simulink model "VB_RIFKF_UWB_INS25"  (R2023a)
settings: Solver=FixedStepAuto  StartTime=0.0  StopTime=500  FixedStep=0.01  RelTol=1e-3
InitFcn:
  | resilient_initNavigation1216;
  | init_param;
  | param_bias;
undefined symbols (not defined in the file or in its folder): dt, g0, gam0_rad, ISUS_flag, lp_GPS_sample_time, lp_Lidar_knoise, lp_Lidar_max, lp_Lidar_min, lp_Lidar_sample_time, lp_Lidar_seed, lp_UWB_knoise, lp_UWB_sample_time, lp_UWB_seed, lp_UWB_XY_max, lp_UWB_XY_min, magnitude, p, P0, P0_RIEKF, param, pd0, pe0, phi0_rad, pn0, psi, psi0_rad, state_dim, vd0, ve0, vn0
libraries: simulink_extras x108, simulink x89, dspstat3 x74, sharedtransform x61, matrix_library x11, sharedTrackingLibrary x8, aerolibconvert2 x5, aerolibtransform2 x5, dspfactors x3
(part 20 of 29)

== system VB_RIFKF_UWB_INS25/ISUS_RIEKF3/Error State Kalman Filter M4/Extended Kalman Filter M1/Correct M1 ==
  yMeas : Inport  SampleTime=SampleTime
  R : Inport  Port=2  SampleTime=SampleTime
  uMeas : Inport  Port=3  SampleTime=SampleTime
  uBlockOrdering : Inport  Port=4  SampleTime=SampleTime
  H : Inport  Port=5  SampleTime=SampleTime
  pk_1 : Inport  Port=6
  Enable : EnablePort
  Cholesky Factorization : dspfactors/Cholesky Factorization  errmode=Warning
  Correct : MATLAB Function  TreatAsAtomicUnit=on
  Data Store Read : DataStoreRead  DataStoreName=x  IndexOptions=Index vector (dialog)  Indices=1  OutputSizes=1
  Data Store Read1 : DataStoreRead  DataStoreName=P  IndexOptions=Index vector (dialog)  Indices=1  OutputSizes=1
  Data Store Write2 : DataStoreWrite  Commented=on  DataStoreName=x  IndexOptions=Index vector (dialog)  Indices=1  OutputSizes=1
  Data Store Write3 : DataStoreWrite  Commented=on  DataStoreName=P  IndexOptions=Index vector (dialog)  Indices=1  OutputSizes=1
  Data Store WriteP : DataStoreWrite  DataStoreName=P  IndexOptions=Index vector (dialog)  Indices=1  OutputSizes=1
  Data Store WriteX : DataStoreWrite  DataStoreName=x  IndexOptions=Index vector (dialog)  Indices=1  OutputSizes=1
  MATLAB Function : MATLAB Function  TreatAsAtomicUnit=on
  R1 : InportShadow  Port=2  SampleTime=SampleTime
  RegisterSimulinkFcn : S-Function  FunctionName=ekfukfRegisterSimulinkFcn  Parameters=int32(3), 1, pM.HasAdditiveNoise, SampleTime, DataType, SLFcnsToRegister  SFunctionDeploymentMode=off  EnableBusSupport=off
  Scope : Scope
  Subsystem2 : Subsystem
  innovation calculation : Subsystem
  yMeas1 : InportShadow  SampleTime=SampleTime
  yBlockOrdering : Outport  VectorParamsAs1DForOutWhenUnconnected=off
  Sk : Outport  Port=2  VectorParamsAs1DForOutWhenUnconnected=off
  m_innov : Outport  Port=3  VectorParamsAs1DForOutWhenUnconnected=off
  wires:
  MATLAB Function/1(y) -> Subsystem2/1(Pk_1_ISIU)
  Cholesky Factorization/1 -> MATLAB Function/1(u)
  pk_1/1 -> Cholesky Factorization/1
  Correct/2(P) -> Data Store WriteP/1
  Data Store Read1/1 -> Subsystem2/2(Pk_2)
  Subsystem2/1(y1) -> Correct/2("P "), innovation calculation/1(Pk/k_1)
  Data Store Read/1 -> RegisterSimulinkFcn/1, Correct/1(x)
  H/1 -> innovation calculation/5(H)
  innovation calculation/1(Sk) -> Sk/1
  innovation calculation/2(m_innov) -> m_innov/1
  R1/1 -> innovation calculation/4(R)
  yMeas1/1 -> innovation calculation/2(yMeas)
  yMeas/1 -> Correct/3(yMeas), RegisterSimulinkFcn/2, Scope/1
  R/1 -> Correct/4(R), RegisterSimulinkFcn/3
  Correct/1(xNew) -> Data Store WriteX/1, innovation calculation/3(X)
  Correct/3(blockOrdering) -> yBlockOrdering/1
  uBlockOrdering/1 -> Correct/6("blockOrdering ")
  uMeas/1 -> Correct/5(uMeas)

== system VB_RIFKF_UWB_INS25/ISUS_RIEKF3/Error State Kalman Filter M4/Extended Kalman Filter M1/Output ==
  uBlockOrdering : Inport
  Data Store Read : DataStoreRead  DataStoreName=x  IndexOptions=Index vector (dialog)  Indices=1  OutputSizes=1
  Data Store Read1 : DataStoreRead  DataStoreName=P  IndexOptions=Index vector (dialog)  Indices=1  OutputSizes=1
  MATLAB Function : MATLAB Function  TreatAsAtomicUnit=on
  x : Outport  VectorParamsAs1DForOutWhenUnconnected=off
  P : Outport  Port=2  VectorParamsAs1DForOutWhenUnconnected=off
  yBlockOrdering : Outport  Port=3  VectorParamsAs1DForOutWhenUnconnected=off
  wires:
  MATLAB Function/1(P) -> P/1
  Data Store Read1/1 -> MATLAB Function/1(S)
  Data Store Read/1 -> x/1
  uBlockOrdering/1 -> yBlockOrdering/1

== system VB_RIFKF_UWB_INS25/ISUS_RIEKF3/Error State Kalman Filter M4/Extended Kalman Filter M1/Predict ==
  Q : Inport  SampleTime=SampleTime
  uState : Inport  Port=2  SampleTime=SampleTime
  uBlockOrdering : Inport  Port=3  SampleTime=SampleTime
  Data Store Read1 : DataStoreRead  Commented=on  DataStoreName=feedback_flag_18dim  IndexOptions=Index vector (dialog)  Indices=1  OutputSizes=1
  Data Store Write : DataStoreWrite  DataStoreName=P  IndexOptions=Index vector (dialog)  Indices=1  OutputSizes=1
  Data Store Write1 : DataStoreWrite  DataStoreName=x  IndexOptions=Index vector (dialog)  Indices=1  OutputSizes=1
  Data Store WriteX : DataStoreWrite  DataStoreName=x  IndexOptions=Index vector (dialog)  Indices=1  OutputSizes=1
  Data Store ReadP : DataStoreRead  DataStoreName=P  IndexOptions=Index vector (dialog)  Indices=1  OutputSizes=1
  Data Store ReadX : DataStoreRead  DataStoreName=x  IndexOptions=Index vector (dialog)  Indices=1  OutputSizes=1
  If : If  Commented=on  IfExpression=u1 == 1  ShowElse=off
  If Action Subsystem : Subsystem  Commented=on  TreatAsAtomicUnit=on
  Predict : MATLAB Function  TreatAsAtomicUnit=on
  RegisterSimulinkFcn : S-Function  FunctionName=ekfukfRegisterSimulinkFcn  Parameters=int32(2), 0, pS.HasAdditiveNoise, SampleTime, DataType, SLFcnsToRegister  SFunctionDeploymentMode=off  EnableBusSupport=off
  Zero : Constant  Value=zeros(state_dim,1)  OutDataTypeStr=Inherit: Inherit via back propagation
  wires:
  Data Store ReadP/1 -> Predict/2("P ")
  Predict/2(P) -> Data Store Write/1
  Q/1 -> Predict/3(Q), RegisterSimulinkFcn/2
  Predict/1(xNew) -> Data Store WriteX/1
  Data Store ReadX/1 -> Predict/1(x), RegisterSimulinkFcn/1
  uBlockOrdering/1 -> Predict/5(unused)
  uState/1 -> Predict/4(uState)
  Data Store Read1/1 -> If/1
  If/1 -> If Action Subsystem/Action
  Zero/1 -> Data Store Write1/1

== system VB_RIFKF_UWB_INS25/ISUS_RIEKF3/Error State Kalman Filter M4/Extended Kalman Filter M1/innovation calculation ==
  Pk/k_1 : Inport
  yMeas : Inport  Port=2
  X : Inport  Port=3
  R : Inport  Port=4
  H : Inport  Port=5
  Add : Sum
  Add1 : Sum  Inputs=+-
  MATLAB Function : MATLAB Function  TreatAsAtomicUnit=on
  Product : Product  Inputs=3  Multiplication=Matrix(*)
  Product1 : Product  Multiplication=Matrix(*)
  Scope1 : Scope
  Scope2 : Scope
  Transpose : Math  Operator=transpose
  Sk : Outport
  m_innov : Outport  Port=2
  wires:
  MATLAB Function/1(y) -> Product/2
  Product/1 -> Add/1
  Transpose/1 -> Product/3
  R/1 -> Add/2
  Pk/k_1/1 -> MATLAB Function/1(u)
  yMeas/1 -> Add1/1
  H/1 -> Product1/1, Product/1, Transpose/1
  X/1 -> Product1/2, Scope2/1
  Product1/1 -> Add1/2
  Add/1 -> Sk/1  "S"
  Add1/1 -> m_innov/1, Scope1/1

== system VB_RIFKF_UWB_INS25/ISUS_RIEKF3/Error State Kalman Filter M4/Simulink Function - State Transition/Cal Phi ==
  Rbn : Inport
  vn : Inport  Port=2
  pn : Inport  Port=3
  Constant : Constant  Value=dt
  MATLAB Function1 : MATLAB Function  TreatAsAtomicUnit=on
  Reshape : Reshape  OutputDimensionality=Column vector (2-D)
  Reshape1 : Reshape  OutputDimensionality=Column vector (2-D)
  Phi : Outport
  wires:
  Reshape1/1 -> MATLAB Function1/2(pn)
  Reshape/1 -> MATLAB Function1/1(vn)
  pn/1 -> Reshape1/1
  vn/1 -> Reshape/1
  Rbn/1 -> MATLAB Function1/3(Rbn)
  MATLAB Function1/1(Phi) -> Phi/1
  Constant/1 -> MATLAB Function1/4(dt)

== system VB_RIFKF_UWB_INS25/ISUS_RIEKF3/Error State Kalman Filter M4/Simulink Function - State Transition1/Cal Phi ==
  Rbn : Inport
  vn : Inport  Port=2
  pn : Inport  Port=3
  Constant : Constant  Value=dt  OutDataTypeStr=single
  MATLAB Function1 : MATLAB Function  TreatAsAtomicUnit=on
  Reshape : Reshape  OutputDimensionality=Column vector (2-D)
  Reshape1 : Reshape  OutputDimensionality=Column vector (2-D)
  Phi : Outport
  wires:
  Constant/1 -> MATLAB Function1/4(dt)
  MATLAB Function1/1(Phi) -> Phi/1
  Rbn/1 -> MATLAB Function1/3(Rbn)
  vn/1 -> Reshape/1
  pn/1 -> Reshape1/1
  Reshape/1 -> MATLAB Function1/1(vn)
  Reshape1/1 -> MATLAB Function1/2(pn)

== system VB_RIFKF_UWB_INS25/ISUS_RIEKF3/Error State Kalman Filter M4/bak/Simulink Function - GPS Measurements1 ==
  DCM_b_n : Inport
  DynamicMeasurementFcn_Dyn : TriggerPort  TriggerType=function-call  IsSimulinkFunction=on  FunctionName=DynamicMeasurementFcn_Dyn  VariantControl=Variant
  Add : Sum  Commented=on
  Add1 : Sum
  Constant : Constant  Commented=on  Value=dt  OutDataTypeStr=single
  Constant6 : Constant  Value=[zeros(3,3),eye(3),zeros(3,12);zeros(3,15),eye(3)]  OutDataTypeStr=single
  Data Type Conversion6 : DataTypeConversion  Commented=on  OutDataTypeStr=single  SaturateOnIntegerOverflow=off  RndMeth=Floor
  From7 : From  Commented=on  GotoTag=DCM_b_n
  Goto : Goto  Commented=on  GotoTag=DCM_b_n
  MATLAB Function1 : MATLAB Function  Commented=on  TreatAsAtomicUnit=on
  Product : Product  Commented=on  Multiplication=Matrix(*)
  Product1 : Product  Multiplication=Matrix(*)
  x : ArgIn  DisableCoverage=on  OutDataTypeStr=single  PortDimensions=18  ArgumentName=x
  v : ArgIn  DisableCoverage=on  Port=2  OutDataTypeStr=single  PortDimensions=6  ArgumentName=v
  y : ArgOut  DisableCoverage=on  OutDataTypeStr=single  PortDimensions=6  ArgumentName=y
  wires:
  x/1 -> Product1/2
  Constant6/1 -> Product1/1
  Product1/1 -> Add1/1
  v/1 -> Add1/2
  Add1/1 -> y/1
  Data Type Conversion6/1 -> Product/1
  DCM_b_n/1 -> Goto/1
  Constant/1 -> MATLAB Function1/2(dt)
  From7/1 -> MATLAB Function1/1(Cbn)
  MATLAB Function1/1(H) -> Data Type Conversion6/1
  Product/1 -> Add/1

== system VB_RIFKF_UWB_INS25/ISUS_RIEKF3/Error State Kalman Filter M4/bak/Simulink Function - GPS Measurements2 ==
  ZUPTMeasurementFcn2 : TriggerPort  TriggerType=function-call  IsSimulinkFunction=on  FunctionName=ZUPTMeasurementFcn2  VariantControl=Variant
  Add : Sum
  Constant6 : Constant  Value=[zeros(3,3),eye(3),zeros(3,12)]  OutDataTypeStr=single
  Product : Product  Multiplication=Matrix(*)
  x : ArgIn  DisableCoverage=on  OutDataTypeStr=single  PortDimensions=18  ArgumentName=x
  v : ArgIn  DisableCoverage=on  Port=2  OutDataTypeStr=single  PortDimensions=3  ArgumentName=v
  y : ArgOut  DisableCoverage=on  OutDataTypeStr=single  PortDimensions=3  ArgumentName=y
  wires:
  v/1 -> Add/2
  Constant6/1 -> Product/1
  x/1 -> Product/2
  Product/1 -> Add/1
  Add/1 -> y/1

== system VB_RIFKF_UWB_INS25/ISUS_RIEKF3/Error State Kalman Filter M4/bak/Simulink Function - State Transition Jacobian ==
  DCM_b_n : Inport
  vn : Inport  Port=2
  pn : Inport  Port=3
  stateTransitionJacobianFcn_Dyn : TriggerPort  TriggerType=function-call  IsSimulinkFunction=on  FunctionName=stateTransitionJacobianFcn_Dyn  VariantControl=Variant
  Cal Phi1 : Subsystem
  Constant : Constant  Value=0.01  OutDataTypeStr=single
  Data Type Conversion1 : DataTypeConversion  OutDataTypeStr=single  SaturateOnIntegerOverflow=off  RndMeth=Floor
  Data Type Conversion6 : DataTypeConversion  OutDataTypeStr=single  SaturateOnIntegerOverflow=off  RndMeth=Floor
  MATLAB Function1 : MATLAB Function  TreatAsAtomicUnit=on
  Product : Product  Multiplication=Matrix(*)
  Terminator : Terminator
  Terminator1 : Terminator
  Transpose : Math  Operator=transpose
  x : ArgIn  DisableCoverage=on  OutDataTypeStr=single  PortDimensions=15  ArgumentName=x
  w : ArgIn  Port=2  OutDataTypeStr=single  PortDimensions=12  ArgumentName=w
  A : ArgOut  DisableCoverage=on  OutDataTypeStr=single  PortDimensions=[15 15]  ArgumentName=A
  G : ArgOut  Port=2  OutDataTypeStr=single  PortDimensions=[15 12]  ArgumentName=G
  wires:
  Data Type Conversion1/1 -> Product/2
  Product/1 -> G/1
  [pn] -> MATLAB Function1/3(pn)
  [vn] -> MATLAB Function1/2(vn)
  Data Type Conversion6/1 -> A/1, Product/1
  Constant/1 -> MATLAB Function1/4(dt)
  Transpose/1 -> MATLAB Function1/1(Rbn)
  [DCM_b_n] -> Transpose/1
  [DCM_b_n] -> Cal Phi1/1(Rbn)
  [pn] -> Cal Phi1/3(pn)
  [vn] -> Cal Phi1/2(vn)
  vn/1 -> [vn]
  pn/1 -> [pn]
  DCM_b_n/1 -> [DCM_b_n]
  Cal Phi1/1(Phi) -> Data Type Conversion6/1
  w/1 -> Terminator1/1
  x/1 -> Terminator/1
  MATLAB Function1/1(G) -> Data Type Conversion1/1

== system VB_RIFKF_UWB_INS25/ISUS_RIEKF3/INS propogation/Init_PVQ/Horizontal_attitude ==
  note: gamma
  note: fai
  accl_mean_B_m/s_LPF : Inport  PortDimensions=3
  Magn_mean_B_guess_LPF : Inport  Port=2
  Enable : EnablePort
  Add : Sum  Commented=on  Inputs=+-
  Add1 : Sum
  Add2 : Sum
  Asin : Trigonometry  Operator=asin
  Atan2 : Trigonometry  Commented=on  Operator=atan2
  Data Type Conversion : DataTypeConversion  SaturateOnIntegerOverflow=off  RndMeth=Floor
  Deal with zero : Subsystem
  Degrees to Radians : simulink_extras/Transformations/Degrees to Radians  Commented=on
  Degrees to Radians1 : simulink_extras/Transformations/Degrees to Radians
  Demux : Demux  Outputs=3
  Display : Display
  Divide : Product  Inputs=*/  OutDataTypeStr=single
  Gain1 : Gain  Gain=-1
  Gain2 : Gain  Gain=-1
  Magnetic declination : Constant  Commented=on  Value=param.fusion.magDeclDeg  OutDataTypeStr=single
  Magnetic declination1 : Constant  Value=param.control.MagnheadingCorrection  OutDataTypeStr=uint8
  Math Function : Math  Operator=magnitude^2  SignedPower=on
  Mux : Mux  Inputs=3
  Mux1 : Mux  Inputs=3
  Mux3 : Mux  Commented=on  Inputs=3
  Product : Product  Commented=on  Multiplication=Matrix(*)
  Quaternions to Direction Cosine Matrix : sharedtransform/Quaternions to  Direction Cosine Matrix  Commented=on  aMode=aMode
  Radians to Degrees : simulink_extras/Transformations/Radians to Degrees  Commented=on
  Rotation Angles to Quaternions : sharedtransform/Rotation Angles to Quaternions  rotationOrder=ZYX  aMode=aMode
  Rotation Angles to Quaternions1 : sharedtransform/Rotation Angles to Quaternions  Commented=on  rotationOrder=ZYX  aMode=aMode
  Scope : Scope
  Scope1 : Scope
  Selector : Selector  Commented=on  InputPortWidth=3  IndexOptions=Index vector (dialog)  Indices=[2]  OutputSizes=1
  Selector1 : Selector  Commented=on  InputPortWidth=3  IndexOptions=Index vector (dialog)  Indices=[1]  OutputSizes=1
  Sqrt : Sqrt
  Sum of Elements : Sum  Inputs=+
  Switch : Switch  Threshold=0.5  SaturateOnIntegerOverflow=off  InputSameDT=off
  Terminator : Terminator  Commented=on
  Transpose : Math  Commented=on  Operator=transpose  SignedPower=on
  Trigonometric Function1 : Trigonometry  Operator=atan2
  phi0_rad : Constant  Value=phi0_rad  OutDataTypeStr=single
  phi0_rad1 : Constant  Value=gam0_rad  OutDataTypeStr=single
  psi_zero : Constant  Value=psi  OutDataTypeStr=single
  psi_zero1 : Constant  Commented=on  Value=psi  OutDataTypeStr=single
  quat_0 : Outport  PortDimensions=4
  wires:
  Gain2/1 -> Add2/2
  phi0_rad1/1 -> Add2/1
  phi0_rad/1 -> Add1/1
  Asin/1 -> Add1/2
  Radians to Degrees/1 -> Display/1
  Data Type Conversion/1 -> Scope/1
  Switch/1 -> quat_0/1, Scope1/1
  Magnetic declination1/1 -> Switch/2, Data Type Conversion/1
  Degrees to Radians/1 -> Terminator/1
  Degrees to Radians1/1 -> Mux1/1
  Gain1/1 -> Mux/3, Trigonometric Function1/2
  Transpose/1 -> Product/1
  Mux3/1 -> Rotation Angles to Quaternions1/1
  Add/1 -> Mux3/1, Radians to Degrees/1  "psi_calbymag"
  Magnetic declination/1 -> Degrees to Radians/1
  Atan2/1 -> Add/2
  Selector/1 -> Atan2/1  "magE"
  Selector1/1 -> Atan2/2  "magN"
  Product/1 -> Selector1/1, Selector/1  "magNED"
  Magn_mean_B_guess_LPF/1 -> Product/2
  Quaternions to Direction Cosine Matrix/1 -> Transpose/1
  Add2/1 -> Mux1/3, Mux3/3
  Add1/1 -> Mux1/2, Mux3/2
  psi_zero/1 -> Degrees to Radians1/1
  Mux1/1 -> Rotation Angles to Quaternions/1
  Math Function/1 -> Sum of Elements/1
  Mux/1 -> Math Function/1
  Divide/1 -> Asin/1
  Sum of Elements/1 -> Sqrt/1
  Demux/3 -> Gain1/1
  Demux/2 -> Trigonometric Function1/1, Mux/1
  Demux/1 -> Mux/2, Divide/1
  Trigonometric Function1/1 -> Gain2/1
  Deal with zero/1(Out1) -> Divide/2
  Sqrt/1 -> Deal with zero/1(In1)
  accl_mean_B_m/s_LPF/1 -> Demux/1
  Rotation Angles to Quaternions/1 -> Switch/1, Switch/3

== system VB_RIFKF_UWB_INS25/ISUS_RIEKF3/INS propogation/Init_PVQ/Subsystem ==
  data : Inport
  Buffer : Buffer  N=50  V=49  OutputFrames=off
  Buffer1 : Buffer  N=50  V=49  OutputFrames=off
  Buffer2 : Buffer  N=50  V=49  ic=-g0  OutputFrames=off
  Demux : Demux  Outputs=3
  Mean4 : dspstat3/Mean  run=off  reset_popup=None  directionMode=Entire input  dimension=3  roiEnable=off  roiType=Rectangles  roiPortion=Entire ROI  roiOutput=Individual statistics for each ROI  roiFlag=off  roundingMode=Floor  overflowMode=off  outputDataTypeStr=Inherit: Same as accumulator  outputMin=[]  outputMax=[]  outputLastDataTypeStr=Inherit: Same as accumulator
  Mean5 : dspstat3/Mean  run=off  reset_popup=None  directionMode=Entire input  dimension=3  roiEnable=off  roiType=Rectangles  roiPortion=Entire ROI  roiOutput=Individual statistics for each ROI  roiFlag=off  roundingMode=Floor  overflowMode=off  outputDataTypeStr=Inherit: Same as accumulator  outputMin=[]  outputMax=[]  outputLastDataTypeStr=Inherit: Same as accumulator
  Mean6 : dspstat3/Mean  run=off  reset_popup=None  directionMode=Entire input  dimension=3  roiEnable=off  roiType=Rectangles  roiPortion=Entire ROI  roiOutput=Individual statistics for each ROI  roiFlag=off  roundingMode=Floor  overflowMode=off  outputDataTypeStr=Inherit: Same as accumulator  outputMin=[]  outputMax=[]  outputLastDataTypeStr=Inherit: Same as accumulator
  Scope : Scope  NumInputPorts=2
  Vector Concatenate : Concatenate  NumInputs=3
  mean_data : Outport
  wires:
  data/1 -> Demux/1, Scope/1
  Vector Concatenate/1 -> mean_data/1, Scope/2
  Mean4/1 -> Vector Concatenate/1
  Demux/3 -> Buffer2/1
  Buffer1/1 -> Mean5/1  "fby_buff"
  Demux/1 -> Buffer/1
  Buffer2/1 -> Mean6/1  "fbz_buff"
  Mean5/1 -> Vector Concatenate/2
  Buffer/1 -> Mean4/1  "fbx_buff"
  Demux/2 -> Buffer1/1
  Mean6/1 -> Vector Concatenate/3

== system VB_RIFKF_UWB_INS25/ISUS_RIEKF3/INS propogation/Init_PVQ/Subsystem1 ==
  data : Inport
  Buffer : Buffer  N=50  V=49  OutputFrames=off
  Buffer1 : Buffer  N=50  V=49  OutputFrames=off
  Buffer2 : Buffer  N=50  V=49  OutputFrames=off
  Demux : Demux  Outputs=3
  Mean4 : dspstat3/Mean  run=off  reset_popup=None  directionMode=Entire input  dimension=3  roiEnable=off  roiType=Rectangles  roiPortion=Entire ROI  roiOutput=Individual statistics for each ROI  roiFlag=off  roundingMode=Floor  overflowMode=off  outputDataTypeStr=Inherit: Same as accumulator  outputMin=[]  outputMax=[]  outputLastDataTypeStr=Inherit: Same as accumulator
  Mean5 : dspstat3/Mean  run=off  reset_popup=None  directionMode=Entire input  dimension=3  roiEnable=off  roiType=Rectangles  roiPortion=Entire ROI  roiOutput=Individual statistics for each ROI  roiFlag=off  roundingMode=Floor  overflowMode=off  outputDataTypeStr=Inherit: Same as accumulator  outputMin=[]  outputMax=[]  outputLastDataTypeStr=Inherit: Same as accumulator
  Mean6 : dspstat3/Mean  run=off  reset_popup=None  directionMode=Entire input  dimension=3  roiEnable=off  roiType=Rectangles  roiPortion=Entire ROI  roiOutput=Individual statistics for each ROI  roiFlag=off  roundingMode=Floor  overflowMode=off  outputDataTypeStr=Inherit: Same as accumulator  outputMin=[]  outputMax=[]  outputLastDataTypeStr=Inherit: Same as accumulator
  Vector Concatenate : Concatenate  NumInputs=3
  mean_data : Outport
  wires:
  Mean6/1 -> Vector Concatenate/3
  Demux/2 -> Buffer1/1
  Buffer/1 -> Mean4/1  "fbx_buff"
  Mean5/1 -> Vector Concatenate/2
  Buffer2/1 -> Mean6/1  "fbz_buff"
  Demux/1 -> Buffer/1
  Buffer1/1 -> Mean5/1  "fby_buff"
  Demux/3 -> Buffer2/1
  Mean4/1 -> Vector Concatenate/1
  Vector Concatenate/1 -> mean_data/1
  data/1 -> Demux/1

== system VB_RIFKF_UWB_INS25/ISUS_RIEKF3/INS propogation/Init_PVQ/Subsystem2 ==
  Degrees to Radians1 : simulink_extras/Transformations/Degrees to Radians
  Degrees to Radians2 : simulink_extras/Transformations/Degrees to Radians
  Degrees to Radians3 : simulink_extras/Transformations/Degrees to Radians
  Mux : Mux  Inputs=3
  Rotation Angles to Quaternions : sharedtransform/Rotation Angles to Quaternions  rotationOrder=ZYX  aMode=aMode
  phi : Constant  Value=0.11  OutDataTypeStr=single
  psi_zero : Constant  Value=psi  OutDataTypeStr=single
  theta : Constant  Value=1.17  OutDataTypeStr=single
  Quat0 : Outport
  wires:
  Degrees to Radians2/1 -> Mux/3
  Degrees to Radians3/1 -> Mux/2
  psi_zero/1 -> Degrees to Radians1/1
  theta/1 -> Degrees to Radians3/1
  Mux/1 -> Rotation Angles to Quaternions/1
  phi/1 -> Degrees to Radians2/1
  Rotation Angles to Quaternions/1 -> Quat0/1
  Degrees to Radians1/1 -> Mux/1

== system VB_RIFKF_UWB_INS25/ISUS_RIEKF3/INS propogation/accl bias compensation/error compensation1 ==
  dda : Inport
  QGC_init : Inport  Port=2
  Add3 : Sum
  Delay : Delay  DelayLength=1  InitialCondition=zeros(3,1)  ExternalReset=Level hold
      settings: InputPortMap=u0,r5
  da : Outport
  wires:
  Add3/1 -> Delay/1, da/1
  QGC_init/1 -> Delay/2
  dda/1 -> Add3/1
  Delay/1 -> Add3/2

== system VB_RIFKF_UWB_INS25/ISUS_RIEKF3/INS propogation/gyro bias compensation/error compensation ==
  ddg : Inport
  Enable : Inport  Port=2
  QGC_init : Inport  Port=3
  Add3 : Sum
  Delay : Delay  DelayLength=1  InitialCondition=zeros(3,1)  ExternalReset=Level hold
      settings: InputPortMap=u0,r5
  If Action Subsystem1 : Subsystem  TreatAsAtomicUnit=on
  If1 : If  IfExpression=u1 == 1  ShowElse=off
  Scope : Scope
  dg : Outport
  wires:
  QGC_init/1 -> Delay/2
  ddg/1 -> Add3/1
  Add3/1 -> dg/1, Delay/1
  Delay/1 -> Add3/2
  If1/1 -> If Action Subsystem1/Action
  Enable/1 -> If1/1, Scope/1

== system VB_RIFKF_UWB_INS25/ISUS_RIEKF3/INS propogation/vel//pos update/Kinematic Equation ==
  Cbn : Inport
  Ab : Inport  Port=2
  Add : Sum  Inputs=+-
  Add1 : Sum  Inputs=+-
  Constant : Constant  Value=[0 0 -g0]  OutDataTypeStr=single
  Constant1 : Constant  Value=[0 0 -g0]  OutDataTypeStr=single
  Product : Product  Multiplication=Matrix(*)  RndMeth=Zero
  Product1 : Product  Multiplication=Matrix(*)  RndMeth=Zero
  Scope : Scope
  Scope1 : Scope  NumInputPorts=2
  Transpose : Math  Operator=transpose
  An : Outport
  ab_nog : Outport  Port=2
  wires:
  Add1/1 -> ab_nog/1  "ab_nog"
  Product1/1 -> Add1/2  "gb"
  Constant1/1 -> Product1/2  "gn"
  Transpose/1 -> Product1/1  "Cnb"
  Constant/1 -> Add/2
  Product/1 -> Add/1, Scope/1
  Ab/1 -> Scope1/1, Add1/1, Product/2
  Add/1 -> Scope1/2, An/1
  Cbn/1 -> Product/1, Transpose/1

== system VB_RIFKF_UWB_INS25/ISUS_RIEKF3/INS propogation/vel//pos update/pos update ==
  dtheta : Inport
  vel_k : Inport  Port=2
  dp : Inport  Port=3
  QGC_init : Inport  Port=4
  p0 : Inport  Port=5
  Add1 : Sum
  Delay1 : Delay  DelayLength=1  InitialConditionSource=Input port  ExternalReset=Rising
      settings: InputPortMap=u0,r5,p4
  Gain1 : Gain  Gain=dt
  MATLAB Function : MATLAB Function  TreatAsAtomicUnit=on
  Reshape1 : Reshape  OutputDimensionality=Column vector (2-D)
  p_k : Outport
  wires:
  MATLAB Function/1(pos_correct) -> p_k/1, Delay1/1
  Add1/1 -> MATLAB Function/3(pos)
  dp/1 -> MATLAB Function/2(KFState_dp)
  dtheta/1 -> MATLAB Function/1(dtheta)
  vel_k/1 -> Gain1/1
  Gain1/1 -> Add1/1
  Delay1/1 -> Add1/2
  Reshape1/1 -> Delay1/3
  QGC_init/1 -> Delay1/2
  p0/1 -> Reshape1/1

== system VB_RIFKF_UWB_INS25/ISUS_RIEKF3/INS propogation/vel//pos update/vel update ==
  dtheta : Inport
  QGC_init : Inport  Port=2
  An : Inport  Port=3
  KFState_dv : Inport  Port=4
  v0 : Inport  Port=5
  Add : Sum
  Delay : Delay  DelayLength=1  InitialConditionSource=Input port  ExternalReset=Rising
      settings: InputPortMap=u0,r5,p4
  Gain : Gain  Gain=dt
  MATLAB Function : MATLAB Function  TreatAsAtomicUnit=on
  Reshape : Reshape  OutputDimensionality=Column vector (2-D)
  vel_k : Outport
  wires:
  MATLAB Function/1(vel_correct) -> vel_k/1, Delay/1
  Add/1 -> MATLAB Function/3(vel)
  dtheta/1 -> MATLAB Function/1(dtheta)
  KFState_dv/1 -> MATLAB Function/2(KFState_dv)
  Delay/1 -> Add/2
  Gain/1 -> Add/1
  v0/1 -> Reshape/1
  An/1 -> Gain/1
  Reshape/1 -> Delay/3
  QGC_init/1 -> Delay/2

== system VB_RIFKF_UWB_INS25/ISUS_RIEKF3/INS propogation1/Init_PVQ/Horizontal_attitude ==
  note: fai
  note: gamma
  accl_mean_B_m/s_LPF : Inport  PortDimensions=3
  Magn_mean_B_guess_LPF : Inport  Port=2
  Enable : EnablePort
  Add : Sum  Commented=on  Inputs=+-
  Add1 : Sum
  Add2 : Sum
  Asin : Trigonometry  Operator=asin
  Atan2 : Trigonometry  Commented=on  Operator=atan2
  Data Type Conversion : DataTypeConversion  SaturateOnIntegerOverflow=off  RndMeth=Floor
  Deal with zero : Subsystem
  Degrees to Radians : simulink_extras/Transformations/Degrees to Radians  Commented=on
  Degrees to Radians1 : simulink_extras/Transformations/Degrees to Radians
  Demux : Demux  Outputs=3
  Display : Display
  Divide : Product  Inputs=*/  OutDataTypeStr=single
  Gain1 : Gain  Gain=-1
  Gain2 : Gain  Gain=-1
  Magnetic declination : Constant  Commented=on  Value=param.fusion.magDeclDeg  OutDataTypeStr=single
  Magnetic declination1 : Constant  Value=param.control.MagnheadingCorrection  OutDataTypeStr=uint8
  Math Function : Math  Operator=magnitude^2  SignedPower=on
  Mux : Mux  Inputs=3
  Mux1 : Mux  Inputs=3
  Mux3 : Mux  Commented=on  Inputs=3
  Product : Product  Commented=on  Multiplication=Matrix(*)
  Quaternions to Direction Cosine Matrix : sharedtransform/Quaternions to  Direction Cosine Matrix  Commented=on  aMode=aMode
  Radians to Degrees : simulink_extras/Transformations/Radians to Degrees  Commented=on
  Rotation Angles to Quaternions : sharedtransform/Rotation Angles to Quaternions  rotationOrder=ZYX  aMode=aMode
  Rotation Angles to Quaternions1 : sharedtransform/Rotation Angles to Quaternions  Commented=on  rotationOrder=ZYX  aMode=aMode
  Scope : Scope
  Scope1 : Scope
  Selector : Selector  Commented=on  InputPortWidth=3  IndexOptions=Index vector (dialog)  Indices=[2]  OutputSizes=1
  Selector1 : Selector  Commented=on  InputPortWidth=3  IndexOptions=Index vector (dialog)  Indices=[1]  OutputSizes=1
  Sqrt : Sqrt
  Sum of Elements : Sum  Inputs=+
  Switch : Switch  Threshold=0.5  SaturateOnIntegerOverflow=off  InputSameDT=off
  Terminator : Terminator  Commented=on
  Transpose : Math  Commented=on  Operator=transpose  SignedPower=on
  Trigonometric Function1 : Trigonometry  Operator=atan2
  phi0_rad : Constant  Value=phi0_rad  OutDataTypeStr=single
  phi0_rad1 : Constant  Value=gam0_rad  OutDataTypeStr=single
  psi_zero : Constant  Value=psi  OutDataTypeStr=single
  psi_zero1 : Constant  Commented=on  Value=psi  OutDataTypeStr=single
  quat_0 : Outport  PortDimensions=4
  wires:
  Rotation Angles to Quaternions/1 -> Switch/3, Switch/1
  accl_mean_B_m/s_LPF/1 -> Demux/1
  Sqrt/1 -> Deal with zero/1(In1)
  Deal with zero/1(Out1) -> Divide/2
  Trigonometric Function1/1 -> Gain2/1
  Demux/1 -> Divide/1, Mux/2
  Demux/2 -> Mux/1, Trigonometric Function1/1
  Demux/3 -> Gain1/1
  Sum of Elements/1 -> Sqrt/1
  Divide/1 -> Asin/1
  Mux/1 -> Math Function/1
  Math Function/1 -> Sum of Elements/1
  Mux1/1 -> Rotation Angles to Quaternions/1
  psi_zero/1 -> Degrees to Radians1/1
  Add1/1 -> Mux3/2, Mux1/2
  Add2/1 -> Mux3/3, Mux1/3
  Quaternions to Direction Cosine Matrix/1 -> Transpose/1
  Magn_mean_B_guess_LPF/1 -> Product/2
  Product/1 -> Selector/1, Selector1/1  "magNED"
  Selector1/1 -> Atan2/2  "magN"
  Selector/1 -> Atan2/1  "magE"
  Atan2/1 -> Add/2
  Magnetic declination/1 -> Degrees to Radians/1
  Add/1 -> Radians to Degrees/1, Mux3/1  "psi_calbymag"
  Mux3/1 -> Rotation Angles to Quaternions1/1
  Transpose/1 -> Product/1
  Gain1/1 -> Trigonometric Function1/2, Mux/3
  Degrees to Radians1/1 -> Mux1/1
  Degrees to Radians/1 -> Terminator/1
  Magnetic declination1/1 -> Data Type Conversion/1, Switch/2
  Switch/1 -> Scope1/1, quat_0/1
  Data Type Conversion/1 -> Scope/1
  Radians to Degrees/1 -> Display/1
  Asin/1 -> Add1/2
  phi0_rad/1 -> Add1/1
  phi0_rad1/1 -> Add2/1
  Gain2/1 -> Add2/2

== system VB_RIFKF_UWB_INS25/ISUS_RIEKF3/INS propogation1/Init_PVQ/Subsystem ==
  data : Inport
  Buffer : Buffer  N=50  V=49  OutputFrames=off
  Buffer1 : Buffer  N=50  V=49  OutputFrames=off
  Buffer2 : Buffer  N=50  V=49  ic=-g0  OutputFrames=off
  Demux : Demux  Outputs=3
  Mean4 : dspstat3/Mean  run=off  reset_popup=None  directionMode=Entire input  dimension=3  roiEnable=off  roiType=Rectangles  roiPortion=Entire ROI  roiOutput=Individual statistics for each ROI  roiFlag=off  roundingMode=Floor  overflowMode=off  outputDataTypeStr=Inherit: Same as accumulator  outputMin=[]  outputMax=[]  outputLastDataTypeStr=Inherit: Same as accumulator
  Mean5 : dspstat3/Mean  run=off  reset_popup=None  directionMode=Entire input  dimension=3  roiEnable=off  roiType=Rectangles  roiPortion=Entire ROI  roiOutput=Individual statistics for each ROI  roiFlag=off  roundingMode=Floor  overflowMode=off  outputDataTypeStr=Inherit: Same as accumulator  outputMin=[]  outputMax=[]  outputLastDataTypeStr=Inherit: Same as accumulator
  Mean6 : dspstat3/Mean  run=off  reset_popup=None  directionMode=Entire input  dimension=3  roiEnable=off  roiType=Rectangles  roiPortion=Entire ROI  roiOutput=Individual statistics for each ROI  roiFlag=off  roundingMode=Floor  overflowMode=off  outputDataTypeStr=Inherit: Same as accumulator  outputMin=[]  outputMax=[]  outputLastDataTypeStr=Inherit: Same as accumulator
  Scope : Scope  NumInputPorts=2
  Vector Concatenate : Concatenate  NumInputs=3
  mean_data : Outport
  wires:
  Mean6/1 -> Vector Concatenate/3
  Demux/2 -> Buffer1/1
  Buffer/1 -> Mean4/1  "fbx_buff"
  Mean5/1 -> Vector Concatenate/2
  Buffer2/1 -> Mean6/1  "fbz_buff"
  Demux/1 -> Buffer/1
  Buffer1/1 -> Mean5/1  "fby_buff"
  Demux/3 -> Buffer2/1
  Mean4/1 -> Vector Concatenate/1
  Vector Concatenate/1 -> Scope/2, mean_data/1
  data/1 -> Scope/1, Demux/1

== system VB_RIFKF_UWB_INS25/ISUS_RIEKF3/INS propogation1/Init_PVQ/Subsystem1 ==
  data : Inport
  Buffer : Buffer  N=50  V=49  OutputFrames=off
  Buffer1 : Buffer  N=50  V=49  OutputFrames=off
  Buffer2 : Buffer  N=50  V=49  OutputFrames=off
  Demux : Demux  Outputs=3
  Mean4 : dspstat3/Mean  run=off  reset_popup=None  directionMode=Entire input  dimension=3  roiEnable=off  roiType=Rectangles  roiPortion=Entire ROI  roiOutput=Individual statistics for each ROI  roiFlag=off  roundingMode=Floor  overflowMode=off  outputDataTypeStr=Inherit: Same as accumulator  outputMin=[]  outputMax=[]  outputLastDataTypeStr=Inherit: Same as accumulator
  Mean5 : dspstat3/Mean  run=off  reset_popup=None  directionMode=Entire input  dimension=3  roiEnable=off  roiType=Rectangles  roiPortion=Entire ROI  roiOutput=Individual statistics for each ROI  roiFlag=off  roundingMode=Floor  overflowMode=off  outputDataTypeStr=Inherit: Same as accumulator  outputMin=[]  outputMax=[]  outputLastDataTypeStr=Inherit: Same as accumulator
  Mean6 : dspstat3/Mean  run=off  reset_popup=None  directionMode=Entire input  dimension=3  roiEnable=off  roiType=Rectangles  roiPortion=Entire ROI  roiOutput=Individual statistics for each ROI  roiFlag=off  roundingMode=Floor  overflowMode=off  outputDataTypeStr=Inherit: Same as accumulator  outputMin=[]  outputMax=[]  outputLastDataTypeStr=Inherit: Same as accumulator
  Vector Concatenate : Concatenate  NumInputs=3
  mean_data : Outport
  wires:
  data/1 -> Demux/1
  Vector Concatenate/1 -> mean_data/1
  Mean4/1 -> Vector Concatenate/1
  Demux/3 -> Buffer2/1
  Buffer1/1 -> Mean5/1  "fby_buff"
  Demux/1 -> Buffer/1
  Buffer2/1 -> Mean6/1  "fbz_buff"
  Mean5/1 -> Vector Concatenate/2
  Buffer/1 -> Mean4/1  "fbx_buff"
  Demux/2 -> Buffer1/1
  Mean6/1 -> Vector Concatenate/3

== system VB_RIFKF_UWB_INS25/ISUS_RIEKF3/INS propogation1/Init_PVQ/Subsystem2 ==
  Degrees to Radians1 : simulink_extras/Transformations/Degrees to Radians
  Degrees to Radians2 : simulink_extras/Transformations/Degrees to Radians
  Degrees to Radians3 : simulink_extras/Transformations/Degrees to Radians
  Mux : Mux  Inputs=3
  Rotation Angles to Quaternions : sharedtransform/Rotation Angles to Quaternions  rotationOrder=ZYX  aMode=aMode
  phi : Constant  Value=0.11  OutDataTypeStr=single
  psi_zero : Constant  Value=psi  OutDataTypeStr=single
  theta : Constant  Value=1.17  OutDataTypeStr=single
  Quat0 : Outport
  wires:
  Degrees to Radians1/1 -> Mux/1
  Rotation Angles to Quaternions/1 -> Quat0/1
  phi/1 -> Degrees to Radians2/1
  Mux/1 -> Rotation Angles to Quaternions/1
  theta/1 -> Degrees to Radians3/1
  psi_zero/1 -> Degrees to Radians1/1
  Degrees to Radians3/1 -> Mux/2
  Degrees to Radians2/1 -> Mux/3

== system VB_RIFKF_UWB_INS25/ISUS_RIEKF3/INS propogation1/accl bias compensation/error compensation1 ==
  dda : Inport
  QGC_init : Inport  Port=2
  Add3 : Sum
  Delay : Delay  DelayLength=1  InitialCondition=zeros(3,1)  ExternalReset=Level hold
      settings: InputPortMap=u0,r5
  da : Outport
  wires:
  Delay/1 -> Add3/2
  dda/1 -> Add3/1
  QGC_init/1 -> Delay/2
  Add3/1 -> da/1, Delay/1

== system VB_RIFKF_UWB_INS25/ISUS_RIEKF3/INS propogation1/gyro bias compensation/error compensation ==
  ddg : Inport
  Enable : Inport  Port=2
  QGC_init : Inport  Port=3
  Add3 : Sum
  Delay : Delay  DelayLength=1  InitialCondition=zeros(3,1)  ExternalReset=Level hold
      settings: InputPortMap=u0,r5
  If Action Subsystem1 : Subsystem  TreatAsAtomicUnit=on
  If1 : If  IfExpression=u1 == 1  ShowElse=off
  Scope : Scope
  dg : Outport
  wires:
  Enable/1 -> Scope/1, If1/1
  If1/1 -> If Action Subsystem1/Action
  Delay/1 -> Add3/2
  Add3/1 -> Delay/1, dg/1
  ddg/1 -> Add3/1
  QGC_init/1 -> Delay/2

== system VB_RIFKF_UWB_INS25/ISUS_RIEKF3/INS propogation1/vel//pos update/Kinematic Equation ==
  Cbn : Inport
  Ab : Inport  Port=2
  Add : Sum  Inputs=+-
  Add1 : Sum  Inputs=+-
  Constant : Constant  Value=[0 0 -g0]  OutDataTypeStr=single
  Constant1 : Constant  Value=[0 0 -g0]  OutDataTypeStr=single
  Product : Product  Multiplication=Matrix(*)  RndMeth=Zero
  Product1 : Product  Multiplication=Matrix(*)  RndMeth=Zero
  Scope : Scope
  Scope1 : Scope  NumInputPorts=2
  Transpose : Math  Operator=transpose
  An : Outport
  ab_nog : Outport  Port=2
  wires:
  Cbn/1 -> Transpose/1, Product/1
  Add/1 -> An/1, Scope1/2
  Ab/1 -> Product/2, Add1/1, Scope1/1
  Product/1 -> Scope/1, Add/1
  Constant/1 -> Add/2
  Transpose/1 -> Product1/1  "Cnb"
  Constant1/1 -> Product1/2  "gn"
  Product1/1 -> Add1/2  "gb"
  Add1/1 -> ab_nog/1  "ab_nog"

== system VB_RIFKF_UWB_INS25/ISUS_RIEKF3/INS propogation1/vel//pos update/pos update ==
  dtheta : Inport
  vel_k : Inport  Port=2
  dp : Inport  Port=3
  QGC_init : Inport  Port=4
  p0 : Inport  Port=5
  Add1 : Sum
  Delay1 : Delay  DelayLength=1  InitialConditionSource=Input port  ExternalReset=Rising
      settings: InputPortMap=u0,r5,p4
  Gain1 : Gain  Gain=dt
  MATLAB Function : MATLAB Function  TreatAsAtomicUnit=on
  Reshape1 : Reshape  OutputDimensionality=Column vector (2-D)
  p_k : Outport
  wires:
  p0/1 -> Reshape1/1
  QGC_init/1 -> Delay1/2
  Reshape1/1 -> Delay1/3
  Delay1/1 -> Add1/2
  Gain1/1 -> Add1/1
  vel_k/1 -> Gain1/1
  dtheta/1 -> MATLAB Function/1(dtheta)
  dp/1 -> MATLAB Function/2(KFState_dp)
  Add1/1 -> MATLAB Function/3(pos)
  MATLAB Function/1(pos_correct) -> Delay1/1, p_k/1

== system VB_RIFKF_UWB_INS25/ISUS_RIEKF3/INS propogation1/vel//pos update/vel update ==
  dtheta : Inport
  QGC_init : Inport  Port=2
  An : Inport  Port=3
  KFState_dv : Inport  Port=4
  v0 : Inport  Port=5
  Add : Sum
  Delay : Delay  DelayLength=1  InitialConditionSource=Input port  ExternalReset=Rising
      settings: InputPortMap=u0,r5,p4
  Gain : Gain  Gain=dt
  MATLAB Function : MATLAB Function  TreatAsAtomicUnit=on
  Reshape : Reshape  OutputDimensionality=Column vector (2-D)
  vel_k : Outport
  wires:
  QGC_init/1 -> Delay/2
  Reshape/1 -> Delay/3
  An/1 -> Gain/1
  v0/1 -> Reshape/1
  Gain/1 -> Add/1
  Delay/1 -> Add/2
  KFState_dv/1 -> MATLAB Function/2(KFState_dv)
  dtheta/1 -> MATLAB Function/1(dtheta)
  Add/1 -> MATLAB Function/3(vel)
  MATLAB Function/1(vel_correct) -> Delay/1, vel_k/1

== system VB_RIFKF_UWB_INS25/ISUS_RIEKF3/INS propogation2/Init_PVQ/Horizontal_attitude ==
  note: gamma
  note: fai
  accl_mean_B_m/s_LPF : Inport  PortDimensions=3
  Magn_mean_B_guess_LPF : Inport  Port=2
  Enable : EnablePort
  Add : Sum  Commented=on  Inputs=+-
  Add1 : Sum
  Add2 : Sum
  Asin : Trigonometry  Operator=asin
  Atan2 : Trigonometry  Commented=on  Operator=atan2
  Data Type Conversion : DataTypeConversion  SaturateOnIntegerOverflow=off  RndMeth=Floor
  Deal with zero : Subsystem
  Degrees to Radians : simulink_extras/Transformations/Degrees to Radians  Commented=on
  Degrees to Radians1 : simulink_extras/Transformations/Degrees to Radians
  Demux : Demux  Outputs=3
  Display : Display
  Divide : Product  Inputs=*/  OutDataTypeStr=single
  Gain1 : Gain  Gain=-1
  Gain2 : Gain  Gain=-1
  Magnetic declination : Constant  Commented=on  Value=param.fusion.magDeclDeg  OutDataTypeStr=single
  Magnetic declination1 : Constant  Value=param.control.MagnheadingCorrection  OutDataTypeStr=uint8
  Math Function : Math  Operator=magnitude^2  SignedPower=on
  Mux : Mux  Inputs=3
  Mux1 : Mux  Inputs=3
  Mux3 : Mux  Commented=on  Inputs=3
  Product : Product  Commented=on  Multiplication=Matrix(*)
  Quaternions to Direction Cosine Matrix : sharedtransform/Quaternions to  Direction Cosine Matrix  Commented=on  aMode=aMode
  Radians to Degrees : simulink_extras/Transformations/Radians to Degrees  Commented=on
  Rotation Angles to Quaternions : sharedtransform/Rotation Angles to Quaternions  rotationOrder=ZYX  aMode=aMode
  Rotation Angles to Quaternions1 : sharedtransform/Rotation Angles to Quaternions  Commented=on  rotationOrder=ZYX  aMode=aMode
  Scope : Scope
  Scope1 : Scope
  Selector : Selector  Commented=on  InputPortWidth=3  IndexOptions=Index vector (dialog)  Indices=[2]  OutputSizes=1
  Selector1 : Selector  Commented=on  InputPortWidth=3  IndexOptions=Index vector (dialog)  Indices=[1]  OutputSizes=1
  Sqrt : Sqrt
  Sum of Elements : Sum  Inputs=+
  Switch : Switch  Threshold=0.5  SaturateOnIntegerOverflow=off  InputSameDT=off
  Terminator : Terminator  Commented=on
  Transpose : Math  Commented=on  Operator=transpose  SignedPower=on
  Trigonometric Function1 : Trigonometry  Operator=atan2
  phi0_rad : Constant  Value=phi0_rad  OutDataTypeStr=single
  phi0_rad1 : Constant  Value=gam0_rad  OutDataTypeStr=single
  psi_zero : Constant  Value=psi  OutDataTypeStr=single
  psi_zero1 : Constant  Commented=on  Value=psi  OutDataTypeStr=single
  quat_0 : Outport  PortDimensions=4
  wires:
  Gain2/1 -> Add2/2
  phi0_rad1/1 -> Add2/1
  phi0_rad/1 -> Add1/1
  Asin/1 -> Add1/2
  Radians to Degrees/1 -> Display/1
  Data Type Conversion/1 -> Scope/1
  Switch/1 -> quat_0/1, Scope1/1
  Magnetic declination1/1 -> Switch/2, Data Type Conversion/1
  Degrees to Radians/1 -> Terminator/1
  Degrees to Radians1/1 -> Mux1/1
  Gain1/1 -> Mux/3, Trigonometric Function1/2
  Transpose/1 -> Product/1
  Mux3/1 -> Rotation Angles to Quaternions1/1
  Add/1 -> Mux3/1, Radians to Degrees/1  "psi_calbymag"
  Magnetic declination/1 -> Degrees to Radians/1
  Atan2/1 -> Add/2
  Selector/1 -> Atan2/1  "magE"
  Selector1/1 -> Atan2/2  "magN"
  Product/1 -> Selector1/1, Selector/1  "magNED"
  Magn_mean_B_guess_LPF/1 -> Product/2
  Quaternions to Direction Cosine Matrix/1 -> Transpose/1
  Add2/1 -> Mux1/3, Mux3/3
  Add1/1 -> Mux1/2, Mux3/2
  psi_zero/1 -> Degrees to Radians1/1
  Mux1/1 -> Rotation Angles to Quaternions/1
  Math Function/1 -> Sum of Elements/1
  Mux/1 -> Math Function/1
  Divide/1 -> Asin/1
  Sum of Elements/1 -> Sqrt/1
  Demux/3 -> Gain1/1
  Demux/2 -> Trigonometric Function1/1, Mux/1
  Demux/1 -> Mux/2, Divide/1
  Trigonometric Function1/1 -> Gain2/1
  Deal with zero/1(Out1) -> Divide/2
  Sqrt/1 -> Deal with zero/1(In1)
  accl_mean_B_m/s_LPF/1 -> Demux/1
  Rotation Angles to Quaternions/1 -> Switch/1, Switch/3

== system VB_RIFKF_UWB_INS25/ISUS_RIEKF3/INS propogation2/Init_PVQ/Subsystem ==
  data : Inport
  Buffer : Buffer  N=50  V=49  OutputFrames=off
  Buffer1 : Buffer  N=50  V=49  OutputFrames=off
  Buffer2 : Buffer  N=50  V=49  ic=-g0  OutputFrames=off
  Demux : Demux  Outputs=3
  Mean4 : dspstat3/Mean  run=off  reset_popup=None  directionMode=Entire input  dimension=3  roiEnable=off  roiType=Rectangles  roiPortion=Entire ROI  roiOutput=Individual statistics for each ROI  roiFlag=off  roundingMode=Floor  overflowMode=off  outputDataTypeStr=Inherit: Same as accumulator  outputMin=[]  outputMax=[]  outputLastDataTypeStr=Inherit: Same as accumulator
  Mean5 : dspstat3/Mean  run=off  reset_popup=None  directionMode=Entire input  dimension=3  roiEnable=off  roiType=Rectangles  roiPortion=Entire ROI  roiOutput=Individual statistics for each ROI  roiFlag=off  roundingMode=Floor  overflowMode=off  outputDataTypeStr=Inherit: Same as accumulator  outputMin=[]  outputMax=[]  outputLastDataTypeStr=Inherit: Same as accumulator
  Mean6 : dspstat3/Mean  run=off  reset_popup=None  directionMode=Entire input  dimension=3  roiEnable=off  roiType=Rectangles  roiPortion=Entire ROI  roiOutput=Individual statistics for each ROI  roiFlag=off  roundingMode=Floor  overflowMode=off  outputDataTypeStr=Inherit: Same as accumulator  outputMin=[]  outputMax=[]  outputLastDataTypeStr=Inherit: Same as accumulator
  Scope : Scope  NumInputPorts=2
  Vector Concatenate : Concatenate  NumInputs=3
  mean_data : Outport
  wires:
  data/1 -> Demux/1, Scope/1
  Vector Concatenate/1 -> mean_data/1, Scope/2
  Mean4/1 -> Vector Concatenate/1
  Demux/3 -> Buffer2/1
  Buffer1/1 -> Mean5/1  "fby_buff"
  Demux/1 -> Buffer/1
  Buffer2/1 -> Mean6/1  "fbz_buff"
  Mean5/1 -> Vector Concatenate/2
  Buffer/1 -> Mean4/1  "fbx_buff"
  Demux/2 -> Buffer1/1
  Mean6/1 -> Vector Concatenate/3

== system VB_RIFKF_UWB_INS25/ISUS_RIEKF3/INS propogation2/Init_PVQ/Subsystem1 ==
  data : Inport
  Buffer : Buffer  N=50  V=49  OutputFrames=off
  Buffer1 : Buffer  N=50  V=49  OutputFrames=off
  Buffer2 : Buffer  N=50  V=49  OutputFrames=off
  Demux : Demux  Outputs=3
  Mean4 : dspstat3/Mean  run=off  reset_popup=None  directionMode=Entire input  dimension=3  roiEnable=off  roiType=Rectangles  roiPortion=Entire ROI  roiOutput=Individual statistics for each ROI  roiFlag=off  roundingMode=Floor  overflowMode=off  outputDataTypeStr=Inherit: Same as accumulator  outputMin=[]  outputMax=[]  outputLastDataTypeStr=Inherit: Same as accumulator
  Mean5 : dspstat3/Mean  run=off  reset_popup=None  directionMode=Entire input  dimension=3  roiEnable=off  roiType=Rectangles  roiPortion=Entire ROI  roiOutput=Individual statistics for each ROI  roiFlag=off  roundingMode=Floor  overflowMode=off  outputDataTypeStr=Inherit: Same as accumulator  outputMin=[]  outputMax=[]  outputLastDataTypeStr=Inherit: Same as accumulator
  Mean6 : dspstat3/Mean  run=off  reset_popup=None  directionMode=Entire input  dimension=3  roiEnable=off  roiType=Rectangles  roiPortion=Entire ROI  roiOutput=Individual statistics for each ROI  roiFlag=off  roundingMode=Floor  overflowMode=off  outputDataTypeStr=Inherit: Same as accumulator  outputMin=[]  outputMax=[]  outputLastDataTypeStr=Inherit: Same as accumulator
  Vector Concatenate : Concatenate  NumInputs=3
  mean_data : Outport
  wires:
  Mean6/1 -> Vector Concatenate/3
  Demux/2 -> Buffer1/1
  Buffer/1 -> Mean4/1  "fbx_buff"
  Mean5/1 -> Vector Concatenate/2
  Buffer2/1 -> Mean6/1  "fbz_buff"
  Demux/1 -> Buffer/1
  Buffer1/1 -> Mean5/1  "fby_buff"
  Demux/3 -> Buffer2/1
  Mean4/1 -> Vector Concatenate/1
  Vector Concatenate/1 -> mean_data/1
  data/1 -> Demux/1

== system VB_RIFKF_UWB_INS25/ISUS_RIEKF3/INS propogation2/Init_PVQ/Subsystem2 ==
  Degrees to Radians1 : simulink_extras/Transformations/Degrees to Radians
  Degrees to Radians2 : simulink_extras/Transformations/Degrees to Radians
  Degrees to Radians3 : simulink_extras/Transformations/Degrees to Radians
  Mux : Mux  Inputs=3
  Rotation Angles to Quaternions : sharedtransform/Rotation Angles to Quaternions  rotationOrder=ZYX  aMode=aMode
  phi : Constant  Value=0.11  OutDataTypeStr=single
  psi_zero : Constant  Value=psi  OutDataTypeStr=single
  theta : Constant  Value=1.17  OutDataTypeStr=single
  Quat0 : Outport
  wires:
  Degrees to Radians2/1 -> Mux/3
  Degrees to Radians3/1 -> Mux/2
  psi_zero/1 -> Degrees to Radians1/1
  theta/1 -> Degrees to Radians3/1
  Mux/1 -> Rotation Angles to Quaternions/1
  phi/1 -> Degrees to Radians2/1
  Rotation Angles to Quaternions/1 -> Quat0/1
  Degrees to Radians1/1 -> Mux/1

== system VB_RIFKF_UWB_INS25/ISUS_RIEKF3/INS propogation2/accl bias compensation/error compensation1 ==
  dda : Inport
  QGC_init : Inport  Port=2
  Add3 : Sum
  Delay : Delay  DelayLength=1  InitialCondition=zeros(3,1)  ExternalReset=Level hold
      settings: InputPortMap=u0,r5
  da : Outport
  wires:
  Add3/1 -> Delay/1, da/1
  QGC_init/1 -> Delay/2
  dda/1 -> Add3/1
  Delay/1 -> Add3/2

== system VB_RIFKF_UWB_INS25/ISUS_RIEKF3/INS propogation2/gyro bias compensation/error compensation ==
  ddg : Inport
  Enable : Inport  Port=2
  QGC_init : Inport  Port=3
  Add3 : Sum
  Delay : Delay  DelayLength=1  InitialCondition=zeros(3,1)  ExternalReset=Level hold
      settings: InputPortMap=u0,r5
  If Action Subsystem1 : Subsystem  TreatAsAtomicUnit=on
  If1 : If  IfExpression=u1 == 1  ShowElse=off
  Scope : Scope
  dg : Outport
  wires:
  QGC_init/1 -> Delay/2
  ddg/1 -> Add3/1
  Add3/1 -> dg/1, Delay/1
  Delay/1 -> Add3/2
  If1/1 -> If Action Subsystem1/Action
  Enable/1 -> If1/1, Scope/1

== system VB_RIFKF_UWB_INS25/ISUS_RIEKF3/INS propogation2/vel//pos update/Kinematic Equation ==
  Cbn : Inport
  Ab : Inport  Port=2
  Add : Sum  Inputs=+-
  Add1 : Sum  Inputs=+-
  Constant : Constant  Value=[0 0 -g0]  OutDataTypeStr=single
  Constant1 : Constant  Value=[0 0 -g0]  OutDataTypeStr=single
  Product : Product  Multiplication=Matrix(*)  RndMeth=Zero
  Product1 : Product  Multiplication=Matrix(*)  RndMeth=Zero
  Scope : Scope
  Scope1 : Scope  NumInputPorts=2
  Transpose : Math  Operator=transpose
  An : Outport
  ab_nog : Outport  Port=2
  wires:
  Add1/1 -> ab_nog/1  "ab_nog"
  Product1/1 -> Add1/2  "gb"
  Constant1/1 -> Product1/2  "gn"
  Transpose/1 -> Product1/1  "Cnb"
  Constant/1 -> Add/2
  Product/1 -> Add/1, Scope/1
  Ab/1 -> Scope1/1, Add1/1, Product/2
  Add/1 -> Scope1/2, An/1
  Cbn/1 -> Product/1, Transpose/1

== system VB_RIFKF_UWB_INS25/ISUS_RIEKF3/INS propogation2/vel//pos update/pos update ==
  dtheta : Inport
  vel_k : Inport  Port=2
  dp : Inport  Port=3
  QGC_init : Inport  Port=4
  p0 : Inport  Port=5
  Add1 : Sum
  Delay1 : Delay  DelayLength=1  InitialConditionSource=Input port  ExternalReset=Rising
      settings: InputPortMap=u0,r5,p4
  Gain1 : Gain  Gain=dt
  MATLAB Function : MATLAB Function  TreatAsAtomicUnit=on
  Reshape1 : Reshape  OutputDimensionality=Column vector (2-D)
  p_k : Outport
  wires:
  MATLAB Function/1(pos_correct) -> p_k/1, Delay1/1
  Add1/1 -> MATLAB Function/3(pos)
  dp/1 -> MATLAB Function/2(KFState_dp)
  dtheta/1 -> MATLAB Function/1(dtheta)
  vel_k/1 -> Gain1/1
  Gain1/1 -> Add1/1
  Delay1/1 -> Add1/2
  Reshape1/1 -> Delay1/3
  QGC_init/1 -> Delay1/2
  p0/1 -> Reshape1/1

== system VB_RIFKF_UWB_INS25/ISUS_RIEKF3/INS propogation2/vel//pos update/vel update ==
  dtheta : Inport
  QGC_init : Inport  Port=2
  An : Inport  Port=3
  KFState_dv : Inport  Port=4
  v0 : Inport  Port=5
  Add : Sum
  Delay : Delay  DelayLength=1  InitialConditionSource=Input port  ExternalReset=Rising
      settings: InputPortMap=u0,r5,p4
  Gain : Gain  Gain=dt
  MATLAB Function : MATLAB Function  TreatAsAtomicUnit=on
  Reshape : Reshape  OutputDimensionality=Column vector (2-D)
  vel_k : Outport
  wires:
  MATLAB Function/1(vel_correct) -> vel_k/1, Delay/1
  Add/1 -> MATLAB Function/3(vel)
  dtheta/1 -> MATLAB Function/1(dtheta)
  KFState_dv/1 -> MATLAB Function/2(KFState_dv)
  Delay/1 -> Add/2
  Gain/1 -> Add/1
  v0/1 -> Reshape/1
  An/1 -> Gain/1
  Reshape/1 -> Delay/3
  QGC_init/1 -> Delay/2
